simulink model "gm_uc3_preparation1_2017"  (R2018a)
settings: Solver=FixedStepDiscrete  StartTime=0.0  StopTime=0.6  FixedStep=2e-5  RelTol=1e-3  EnableMultiTasking=on
libraries: hdlsllib x6, simulink x3
(part 1 of 2)
settings Model: Creator=elahifah16  LastModifiedBy=Talha Rao
settings SolverCC: PositivePriorityOrder=on
settings OptimizationCC: BlockReduction=off  ConditionallyExecuteInputs=off  DefaultUnderspecifiedDataType=single  PassReuseOutputArgsAs=Individual arguments  MaxStackSize=64
settings DebuggingCC: InheritedTsInSrcMsg=none  ParameterTunabilityLossMsg=error  BusObjectLabelMismatch=error
settings HardwareCC: ProdBitPerPointer=32  ProdBitPerSizeT=32  ProdBitPerPtrDiffT=32  ProdLargestAtomicInteger=Long  ProdLargestAtomicFloat=Double  ProdWordSize=32  ProdHWDeviceType=ARM Compatible->ARM Cortex
settings SFSimCC: MATLABDynamicMemAlloc=off
settings RTWCC: SystemTargetFile=ert.tlc  HardwareBoard=Xilinx Zynq-7000 based board  TLCOptions="-aInlineSetEventsForThisBaseRateFcn=TLC_FALSE -aSuppressMultiTaskScheduler=TLC_FALSE  -aRateBasedStepFcn=0"  GenCodeOnly=on  TemplateMakefile=ert_default_tmf  GenerateReport=on  Toolchain=Xilinx Software Development Kit (SDK)  IncludeHyperlinkInReport=on  LaunchReport=on  GenerateTraceInfo=on  GenerateTraceReport=on  GenerateTraceReportSl=on  GenerateTraceReportSf=on  GenerateTraceReportEml=on  GenerateCodeReplacementReport=on
settings CodeAppCC: ForceParamTrailComments=on  IgnoreCustomStorageClasses=off  OperatorAnnotations=on  SimulinkDataObjDesc=on  SFDataObjDesc=on  InsertBlockDesc=on  StateflowObjectComments=on
settings ERTTargetCC: CodeReplacementLibrary=GNU C99 extensions  SupportComplex=off  SupportVariableSizeSignals=on  ExtModeTransport=1  ExtModeMexFile=ext_serial_win32_comm  MultiInstanceErrorCode=None  RootIOFormat=Structure reference

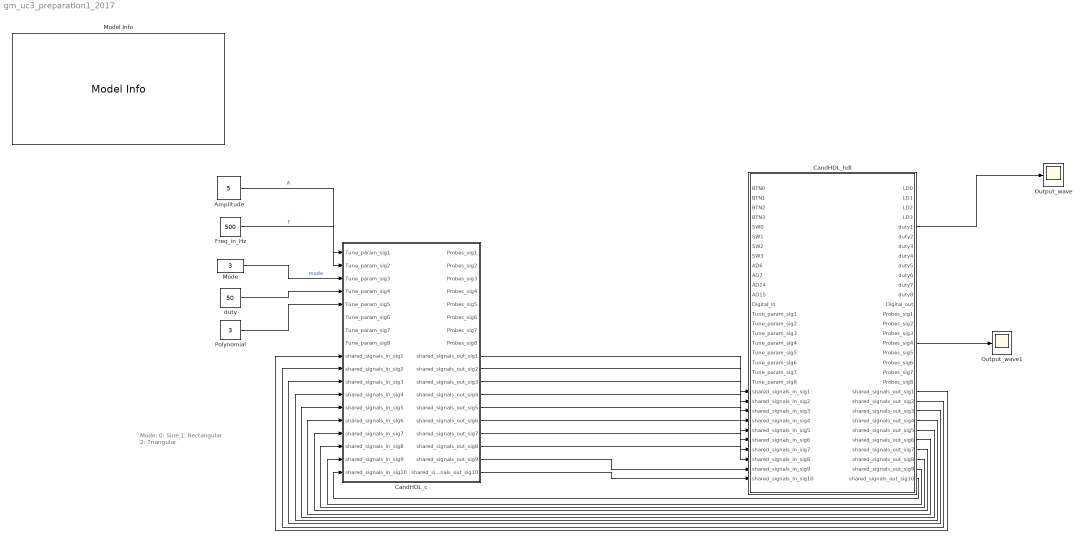
== system gm_uc3_preparation1_2017 ==
  note: Mode:
      | 0: Sine
      | 1: Rectangular
      | 2: Triangular
  Amplitude : Constant  Value=5  OutDataTypeStr=int32
  CandHDL_c : Subsystem  AncestorBlock=code_gen_library/CandHDL_c
  CandHDL_hdl : Subsystem
  Freq_in_Hz : Constant  Value=500  OutDataTypeStr=int32
  Mode : Constant  Value=3  OutDataTypeStr=int32
  Model Info : simulink/Model-Wide Utilities/Model Info  Frame=on  DisplayStringWithTags=|  HorizontalTextAlignment=Left  LeftAlignmentValue=0.02
      | Model Info
      | Creator:       R. Estrada, FH JOANNEUM, 2018
      | Modified by: %<ModifiedBy>
      | Modify Date: %<ModifiedDate>
      | Version:%<ModelVersion>
      | Description:
      | %<Description>
  Output_wave : Scope
  Output_wave1 : Scope
  Polynomial : Constant  Value=3  OutDataTypeStr=int32
  duty : Constant  Value=50  VectorParams1D=off  OutDataTypeStr=int32
  wires:
  CandHDL_hdl/17(Probes_sig4) -> Output_wave1/1
  Mode/1 -> CandHDL_c/3(Tune_param_sig3)  "mode"
  Freq_in_Hz/1 -> CandHDL_c/2(Tune_param_sig2)  "f"
  Polynomial/1 -> CandHDL_c/5(Tune_param_sig5)
  Amplitude/1 -> CandHDL_c/1(Tune_param_sig1)  "A"
  duty/1 -> CandHDL_c/4(Tune_param_sig4)
  CandHDL_hdl/31(shared_signals_out_sig10) -> CandHDL_c/18(shared_signals_in_sig10)
  CandHDL_c/18(shared_signals_out_sig10) -> CandHDL_hdl/31(shared_signals_in_sig10)
  CandHDL_hdl/30(shared_signals_out_sig9) -> CandHDL_c/17(shared_signals_in_sig9)
  CandHDL_c/17(shared_signals_out_sig9) -> CandHDL_hdl/30(shared_signals_in_sig9)
  CandHDL_hdl/29(shared_signals_out_sig8) -> CandHDL_c/16(shared_signals_in_sig8)
  CandHDL_c/16(shared_signals_out_sig8) -> CandHDL_hdl/29(shared_signals_in_sig8)
  CandHDL_hdl/28(shared_signals_out_sig7) -> CandHDL_c/15(shared_signals_in_sig7)
  CandHDL_c/15(shared_signals_out_sig7) -> CandHDL_hdl/28(shared_signals_in_sig7)
  CandHDL_hdl/27(shared_signals_out_sig6) -> CandHDL_c/14(shared_signals_in_sig6)
  CandHDL_c/14(shared_signals_out_sig6) -> CandHDL_hdl/27(shared_signals_in_sig6)
  CandHDL_hdl/26(shared_signals_out_sig5) -> CandHDL_c/13(shared_signals_in_sig5)
  CandHDL_c/13(shared_signals_out_sig5) -> CandHDL_hdl/26(shared_signals_in_sig5)
  CandHDL_hdl/25(shared_signals_out_sig4) -> CandHDL_c/12(shared_signals_in_sig4)
  CandHDL_c/12(shared_signals_out_sig4) -> CandHDL_hdl/25(shared_signals_in_sig4)
  CandHDL_hdl/24(shared_signals_out_sig3) -> CandHDL_c/11(shared_signals_in_sig3)
  CandHDL_c/11(shared_signals_out_sig3) -> CandHDL_hdl/24(shared_signals_in_sig3)
  CandHDL_hdl/23(shared_signals_out_sig2) -> CandHDL_c/10(shared_signals_in_sig2)
  CandHDL_c/10(shared_signals_out_sig2) -> CandHDL_hdl/23(shared_signals_in_sig2)
  CandHDL_hdl/22(shared_signals_out_sig1) -> CandHDL_c/9(shared_signals_in_sig1)
  CandHDL_c/9(shared_signals_out_sig1) -> CandHDL_hdl/22(shared_signals_in_sig1)
  CandHDL_hdl/5(duty1) -> Output_wave/1

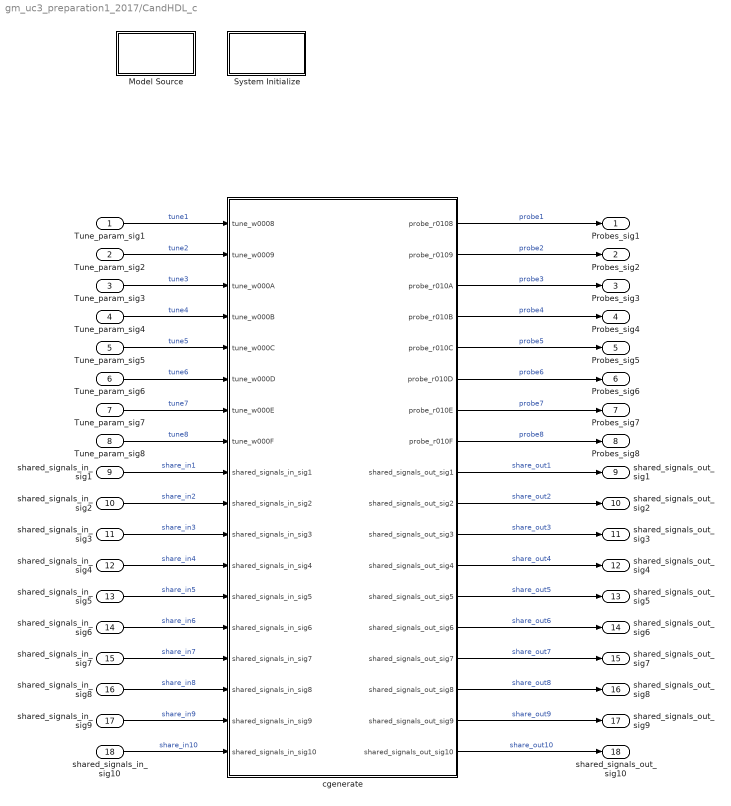
== system gm_uc3_preparation1_2017/CandHDL_c ==
  Tune_param_sig1 : Inport  OutDataTypeStr=int32
  Tune_param_sig2 : Inport  Port=2  OutDataTypeStr=int32
  Tune_param_sig3 : Inport  Port=3  OutDataTypeStr=int32
  Tune_param_sig4 : Inport  Port=4  OutDataTypeStr=int32
  Tune_param_sig5 : Inport  Port=5  OutDataTypeStr=int32
  Tune_param_sig6 : Inport  Port=6  OutDataTypeStr=int32
  Tune_param_sig7 : Inport  Port=7  OutDataTypeStr=int32
  Tune_param_sig8 : Inport  Port=8  OutDataTypeStr=int32
  shared_signals_in_sig1 : Inport  Port=9  OutDataTypeStr=int32
  shared_signals_in_sig2 : Inport  Port=10  OutDataTypeStr=int32
  shared_signals_in_sig3 : Inport  Port=11  OutDataTypeStr=int32
  shared_signals_in_sig4 : Inport  Port=12  OutDataTypeStr=int32
  shared_signals_in_sig5 : Inport  Port=13  OutDataTypeStr=int32
  shared_signals_in_sig6 : Inport  Port=14  OutDataTypeStr=int32
  shared_signals_in_sig7 : Inport  Port=15  OutDataTypeStr=int32
  shared_signals_in_sig8 : Inport  Port=16  OutDataTypeStr=int32
  shared_signals_in_sig9 : Inport  Port=17  OutDataTypeStr=int32
  shared_signals_in_sig10 : Inport  Port=18  OutDataTypeStr=int32
  Model Source : Subsystem  mask(Model Source){ShowInLibBrowser=0}
      mask prompts: ShowInLibBrowser "Simulink:masks:CustCodeMaskParam1_MP"
      settings: CopyFcn=cccopyfcn(gcb)  OpenFcn=ccopenfcn('Model Source')
      mask Help: eval('feval(''rtwprivate'',''rtwhelpview'',''rtw_model_source_block'')');
      mask Display: disp('Model\nSource');
  System Initialize : Subsystem  mask(System Initialize){ShowInLibBrowser=0}
      mask prompts: ShowInLibBrowser "Simulink:masks:CustCodeMaskParam1_MP"
      settings: CopyFcn=cccopyfcn(gcb)  OpenFcn=ccopenfcn('System Initialize Function')
      mask Help: eval('feval(''rtwprivate'',''rtwhelpview'',''rtw_sys_initialize_block'')');
      mask Display: disp('System\nInitialize');
  cgenerate : Subsystem
  Probes_sig1 : Outport  OutDataTypeStr=int32
  Probes_sig2 : Outport  Port=2  OutDataTypeStr=int32
  Probes_sig3 : Outport  Port=3  OutDataTypeStr=int32
  Probes_sig4 : Outport  Port=4  OutDataTypeStr=int32
  Probes_sig5 : Outport  Port=5  OutDataTypeStr=int32
  Probes_sig6 : Outport  Port=6  OutDataTypeStr=int32
  Probes_sig7 : Outport  Port=7  OutDataTypeStr=int32
  Probes_sig8 : Outport  Port=8  OutDataTypeStr=int32
  shared_signals_out_sig1 : Outport  Port=9  OutDataTypeStr=int32
  shared_signals_out_sig2 : Outport  Port=10  OutDataTypeStr=int32
  shared_signals_out_sig3 : Outport  Port=11  OutDataTypeStr=int32
  shared_signals_out_sig4 : Outport  Port=12  OutDataTypeStr=int32
  shared_signals_out_sig5 : Outport  Port=13  OutDataTypeStr=int32
  shared_signals_out_sig6 : Outport  Port=14  OutDataTypeStr=int32
  shared_signals_out_sig7 : Outport  Port=15  OutDataTypeStr=int32
  shared_signals_out_sig8 : Outport  Port=16  OutDataTypeStr=int32
  shared_signals_out_sig9 : Outport  Port=17  OutDataTypeStr=int32
  shared_signals_out_sig10 : Outport  Port=18  OutDataTypeStr=int32
  wires:
  cgenerate/18(shared_signals_out_sig10) -> shared_signals_out_sig10/1  "share_out10"
  cgenerate/17(shared_signals_out_sig9) -> shared_signals_out_sig9/1  "share_out9"
  cgenerate/16(shared_signals_out_sig8) -> shared_signals_out_sig8/1  "share_out8"
  cgenerate/15(shared_signals_out_sig7) -> shared_signals_out_sig7/1  "share_out7"
  cgenerate/14(shared_signals_out_sig6) -> shared_signals_out_sig6/1  "share_out6"
  cgenerate/13(shared_signals_out_sig5) -> shared_signals_out_sig5/1  "share_out5"
  cgenerate/12(shared_signals_out_sig4) -> shared_signals_out_sig4/1  "share_out4"
  cgenerate/11(shared_signals_out_sig3) -> shared_signals_out_sig3/1  "share_out3"
  cgenerate/10(shared_signals_out_sig2) -> shared_signals_out_sig2/1  "share_out2"
  cgenerate/9(shared_signals_out_sig1) -> shared_signals_out_sig1/1  "share_out1"
  shared_signals_in_sig10/1 -> cgenerate/18(shared_signals_in_sig10)  "share_in10"
  shared_signals_in_sig9/1 -> cgenerate/17(shared_signals_in_sig9)  "share_in9"
  shared_signals_in_sig8/1 -> cgenerate/16(shared_signals_in_sig8)  "share_in8"
  shared_signals_in_sig7/1 -> cgenerate/15(shared_signals_in_sig7)  "share_in7"
  shared_signals_in_sig6/1 -> cgenerate/14(shared_signals_in_sig6)  "share_in6"
  shared_signals_in_sig5/1 -> cgenerate/13(shared_signals_in_sig5)  "share_in5"
  shared_signals_in_sig4/1 -> cgenerate/12(shared_signals_in_sig4)  "share_in4"
  shared_signals_in_sig3/1 -> cgenerate/11(shared_signals_in_sig3)  "share_in3"
  shared_signals_in_sig2/1 -> cgenerate/10(shared_signals_in_sig2)  "share_in2"
  shared_signals_in_sig1/1 -> cgenerate/9(shared_signals_in_sig1)  "share_in1"
  Tune_param_sig8/1 -> cgenerate/8(tune_w000F)  "tune8"
  Tune_param_sig7/1 -> cgenerate/7(tune_w000E)  "tune7"
  Tune_param_sig6/1 -> cgenerate/6(tune_w000D)  "tune6"
  Tune_param_sig5/1 -> cgenerate/5(tune_w000C)  "tune5"
  Tune_param_sig4/1 -> cgenerate/4(tune_w000B)  "tune4"
  Tune_param_sig3/1 -> cgenerate/3(tune_w000A)  "tune3"
  Tune_param_sig2/1 -> cgenerate/2(tune_w0009)  "tune2"
  Tune_param_sig1/1 -> cgenerate/1(tune_w0008)  "tune1"
  cgenerate/8(probe_r010F) -> Probes_sig8/1  "probe8"
  cgenerate/7(probe_r010E) -> Probes_sig7/1  "probe7"
  cgenerate/6(probe_r010D) -> Probes_sig6/1  "probe6"
  cgenerate/5(probe_r010C) -> Probes_sig5/1  "probe5"
  cgenerate/4(probe_r010B) -> Probes_sig4/1  "probe4"
  cgenerate/3(probe_r010A) -> Probes_sig3/1  "probe3"
  cgenerate/2(probe_r0109) -> Probes_sig2/1  "probe2"
  cgenerate/1(probe_r0108) -> Probes_sig1/1  "probe1"

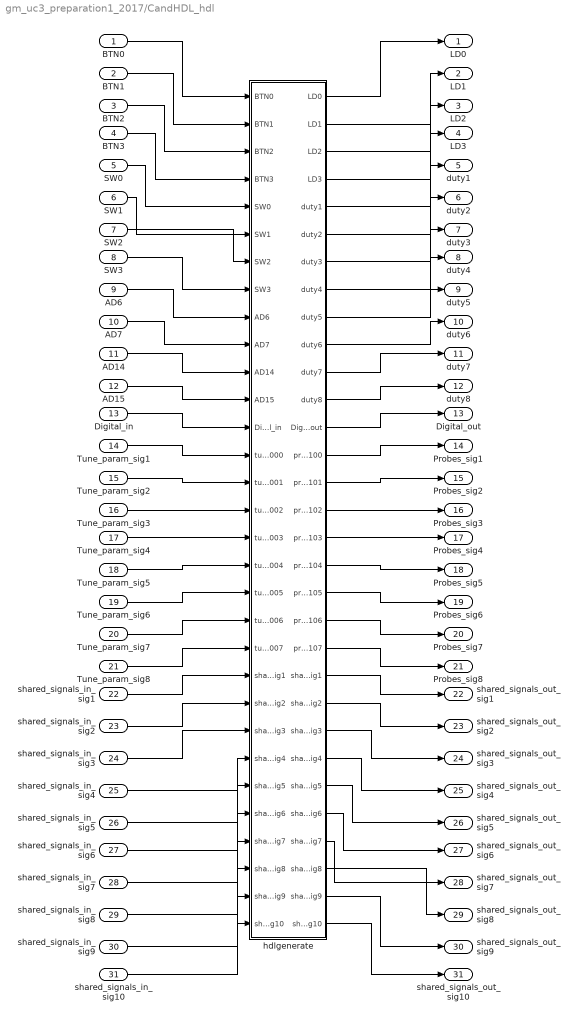
== system gm_uc3_preparation1_2017/CandHDL_hdl ==
  BTN0 : Inport  OutDataTypeStr=boolean  PortDimensions=1
  BTN1 : Inport  Port=2  OutDataTypeStr=boolean  PortDimensions=1
  BTN2 : Inport  Port=3  OutDataTypeStr=boolean  PortDimensions=1
  BTN3 : Inport  Port=4  OutDataTypeStr=boolean  PortDimensions=1
  SW0 : Inport  Port=5  OutDataTypeStr=boolean  PortDimensions=1
  SW1 : Inport  Port=6  OutDataTypeStr=boolean  PortDimensions=1
  SW2 : Inport  Port=7  OutDataTypeStr=boolean  PortDimensions=1
  SW3 : Inport  Port=8  OutDataTypeStr=boolean  PortDimensions=1
  AD6 : Inport  Port=9  OutDataTypeStr=uint16  PortDimensions=1
  AD7 : Inport  Port=10  OutDataTypeStr=uint16  PortDimensions=1
  AD14 : Inport  Port=11  OutDataTypeStr=uint16  PortDimensions=1
  AD15 : Inport  Port=12  OutDataTypeStr=uint16  PortDimensions=1
  Digital_in : Inport  Port=13  OutDataTypeStr=uint8  PortDimensions=1
  Tune_param_sig1 : Inport  Port=14  OutDataTypeStr=int32  PortDimensions=1
  Tune_param_sig2 : Inport  Port=15  OutDataTypeStr=int32  PortDimensions=1
  Tune_param_sig3 : Inport  Port=16  OutDataTypeStr=int32  PortDimensions=1
  Tune_param_sig4 : Inport  Port=17  OutDataTypeStr=int32  PortDimensions=1
  Tune_param_sig5 : Inport  Port=18  OutDataTypeStr=int32  PortDimensions=1
  Tune_param_sig6 : Inport  Port=19  OutDataTypeStr=int32  PortDimensions=1
  Tune_param_sig7 : Inport  Port=20  OutDataTypeStr=int32  PortDimensions=1
  Tune_param_sig8 : Inport  Port=21  OutDataTypeStr=int32  PortDimensions=1
  shared_signals_in_sig1 : Inport  Port=22  OutDataTypeStr=int32  PortDimensions=1
  shared_signals_in_sig2 : Inport  Port=23  OutDataTypeStr=int32  PortDimensions=1  SampleTime=2e-05
  shared_signals_in_sig3 : Inport  Port=24  OutDataTypeStr=int32  PortDimensions=1  SampleTime=2e-05
  shared_signals_in_sig4 : Inport  Port=25  OutDataTypeStr=int32  PortDimensions=1  SampleTime=2e-05
  shared_signals_in_sig5 : Inport  Port=26  OutDataTypeStr=int32  PortDimensions=1  SampleTime=2e-05
  shared_signals_in_sig6 : Inport  Port=27  OutDataTypeStr=int32  PortDimensions=1  SampleTime=2e-05
  shared_signals_in_sig7 : Inport  Port=28  OutDataTypeStr=int32  PortDimensions=1
  shared_signals_in_sig8 : Inport  Port=29  OutDataTypeStr=int32  PortDimensions=1  SampleTime=2e-05
  shared_signals_in_sig9 : Inport  Port=30  OutDataTypeStr=int32  PortDimensions=1
  shared_signals_in_sig10 : Inport  Port=31  OutDataTypeStr=int32  PortDimensions=1
  hdlgenerate : Subsystem
  LD0 : Outport  OutDataTypeStr=boolean
  LD1 : Outport  Port=2  OutDataTypeStr=boolean
  LD2 : Outport  Port=3  OutDataTypeStr=boolean
  LD3 : Outport  Port=4  OutDataTypeStr=boolean
  duty1 : Outport  Port=5  OutDataTypeStr=uint16
  duty2 : Outport  Port=6  OutDataTypeStr=uint16
  duty3 : Outport  Port=7  OutDataTypeStr=uint16
  duty4 : Outport  Port=8  OutDataTypeStr=uint16
  duty5 : Outport  Port=9  OutDataTypeStr=uint16
  duty6 : Outport  Port=10  OutDataTypeStr=uint16
  duty7 : Outport  Port=11  OutDataTypeStr=uint16
  duty8 : Outport  Port=12  OutDataTypeStr=uint16
  Digital_out : Outport  Port=13  OutDataTypeStr=uint8
  Probes_sig1 : Outport  Port=14  OutDataTypeStr=int32
  Probes_sig2 : Outport  Port=15  OutDataTypeStr=int32
  Probes_sig3 : Outport  Port=16  OutDataTypeStr=int32
  Probes_sig4 : Outport  Port=17  OutDataTypeStr=int32
  Probes_sig5 : Outport  Port=18  OutDataTypeStr=int32
  Probes_sig6 : Outport  Port=19  OutDataTypeStr=int32
  Probes_sig7 : Outport  Port=20  OutDataTypeStr=int32
  Probes_sig8 : Outport  Port=21  OutDataTypeStr=int32
  shared_signals_out_sig1 : Outport  Port=22  OutDataTypeStr=int32
  shared_signals_out_sig2 : Outport  Port=23  OutDataTypeStr=int32
  shared_signals_out_sig3 : Outport  Port=24  OutDataTypeStr=int32
  shared_signals_out_sig4 : Outport  Port=25  OutDataTypeStr=int32
  shared_signals_out_sig5 : Outport  Port=26  OutDataTypeStr=int32
  shared_signals_out_sig6 : Outport  Port=27  OutDataTypeStr=int32
  shared_signals_out_sig7 : Outport  Port=28  OutDataTypeStr=int32
  shared_signals_out_sig8 : Outport  Port=29  OutDataTypeStr=int32
  shared_signals_out_sig9 : Outport  Port=30  OutDataTypeStr=int32
  shared_signals_out_sig10 : Outport  Port=31  OutDataTypeStr=int32
  wires:
  BTN0/1 -> hdlgenerate/1(BTN0)
  BTN1/1 -> hdlgenerate/2(BTN1)
  BTN2/1 -> hdlgenerate/3(BTN2)
  BTN3/1 -> hdlgenerate/4(BTN3)
  SW0/1 -> hdlgenerate/5(SW0)
  SW1/1 -> hdlgenerate/6(SW1)
  SW2/1 -> hdlgenerate/7(SW2)
  SW3/1 -> hdlgenerate/8(SW3)
  AD6/1 -> hdlgenerate/9(AD6)
  AD7/1 -> hdlgenerate/10(AD7)
  AD14/1 -> hdlgenerate/11(AD14)
  AD15/1 -> hdlgenerate/12(AD15)
  Digital_in/1 -> hdlgenerate/13(Digital_in)
  Tune_param_sig1/1 -> hdlgenerate/14(tune_w0000)
  Tune_param_sig2/1 -> hdlgenerate/15(tune_w0001)
  Tune_param_sig3/1 -> hdlgenerate/16(tune_w0002)
  Tune_param_sig4/1 -> hdlgenerate/17(tune_w0003)
  Tune_param_sig5/1 -> hdlgenerate/18(tune_w0004)
  Tune_param_sig6/1 -> hdlgenerate/19(tune_w0005)
  Tune_param_sig7/1 -> hdlgenerate/20(tune_w0006)
  Tune_param_sig8/1 -> hdlgenerate/21(tune_w0007)
  shared_signals_in_sig1/1 -> hdlgenerate/22(shared_signals_in_sig1)
  shared_signals_in_sig2/1 -> hdlgenerate/23(shared_signals_in_sig2)
  shared_signals_in_sig3/1 -> hdlgenerate/24(shared_signals_in_sig3)
  shared_signals_in_sig4/1 -> hdlgenerate/25(shared_signals_in_sig4)
  shared_signals_in_sig5/1 -> hdlgenerate/26(shared_signals_in_sig5)
  shared_signals_in_sig6/1 -> hdlgenerate/27(shared_signals_in_sig6)
  shared_signals_in_sig7/1 -> hdlgenerate/28(shared_signals_in_sig7)
  shared_signals_in_sig8/1 -> hdlgenerate/29(shared_signals_in_sig8)
  shared_signals_in_sig9/1 -> hdlgenerate/30(shared_signals_in_sig9)
  shared_signals_in_sig10/1 -> hdlgenerate/31(shared_signals_in_sig10)
  hdlgenerate/1(LD0) -> LD0/1
  hdlgenerate/2(LD1) -> LD1/1
  hdlgenerate/3(LD2) -> LD2/1
  hdlgenerate/4(LD3) -> LD3/1
  hdlgenerate/5(duty1) -> duty1/1
  hdlgenerate/6(duty2) -> duty2/1
  hdlgenerate/7(duty3) -> duty3/1
  hdlgenerate/8(duty4) -> duty4/1
  hdlgenerate/9(duty5) -> duty5/1
  hdlgenerate/10(duty6) -> duty6/1
  hdlgenerate/11(duty7) -> duty7/1
  hdlgenerate/12(duty8) -> duty8/1
  hdlgenerate/13(Digital_out) -> Digital_out/1
  hdlgenerate/14(probe_r0100) -> Probes_sig1/1
  hdlgenerate/15(probe_r0101) -> Probes_sig2/1
  hdlgenerate/16(probe_r0102) -> Probes_sig3/1
  hdlgenerate/17(probe_r0103) -> Probes_sig4/1
  hdlgenerate/18(probe_r0104) -> Probes_sig5/1
  hdlgenerate/19(probe_r0105) -> Probes_sig6/1
  hdlgenerate/20(probe_r0106) -> Probes_sig7/1
  hdlgenerate/21(probe_r0107) -> Probes_sig8/1
  hdlgenerate/22(shared_signals_out_sig1) -> shared_signals_out_sig1/1
  hdlgenerate/23(shared_signals_out_sig2) -> shared_signals_out_sig2/1
  hdlgenerate/24(shared_signals_out_sig3) -> shared_signals_out_sig3/1
  hdlgenerate/25(shared_signals_out_sig4) -> shared_signals_out_sig4/1
  hdlgenerate/26(shared_signals_out_sig5) -> shared_signals_out_sig5/1
  hdlgenerate/27(shared_signals_out_sig6) -> shared_signals_out_sig6/1
  hdlgenerate/28(shared_signals_out_sig7) -> shared_signals_out_sig7/1
  hdlgenerate/29(shared_signals_out_sig8) -> shared_signals_out_sig8/1
  hdlgenerate/30(shared_signals_out_sig9) -> shared_signals_out_sig9/1
  hdlgenerate/31(shared_signals_out_sig10) -> shared_signals_out_sig10/1

== system gm_uc3_preparation1_2017/CandHDL_c/Model Source ==

== system gm_uc3_preparation1_2017/CandHDL_c/System Initialize ==

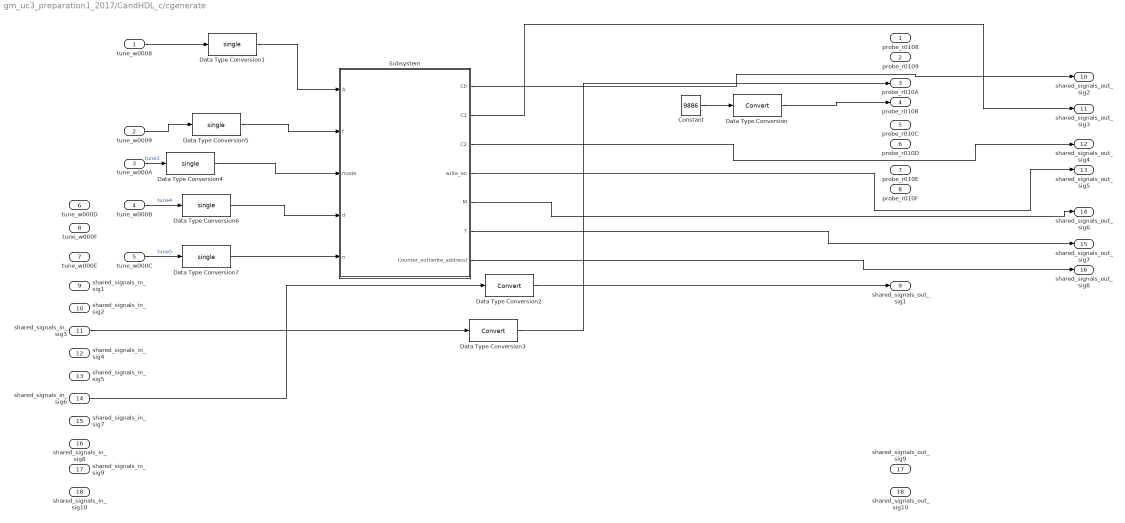
== system gm_uc3_preparation1_2017/CandHDL_c/cgenerate ==
  tune_w0008 : Inport  OutDataTypeStr=int32
  tune_w0009 : Inport  Port=2  OutDataTypeStr=int32
  tune_w000A : Inport  Port=3  OutDataTypeStr=int32
  tune_w000B : Inport  Port=4  OutDataTypeStr=int32
  tune_w000C : Inport  Port=5  OutDataTypeStr=int32
  tune_w000D : Inport  Port=6  OutDataTypeStr=int32
  tune_w000E : Inport  Port=7  OutDataTypeStr=int32
  tune_w000F : Inport  Port=8  OutDataTypeStr=int32
  shared_signals_in_sig1 : Inport  Port=9  OutDataTypeStr=int32
  shared_signals_in_sig2 : Inport  Port=10  OutDataTypeStr=int32
  shared_signals_in_sig3 : Inport  Port=11  OutDataTypeStr=int32
  shared_signals_in_sig4 : Inport  Port=12  OutDataTypeStr=int32
  shared_signals_in_sig5 : Inport  Port=13  OutDataTypeStr=int32
  shared_signals_in_sig6 : Inport  Port=14  OutDataTypeStr=int32
  shared_signals_in_sig7 : Inport  Port=15  OutDataTypeStr=int32
  shared_signals_in_sig8 : Inport  Port=16  OutDataTypeStr=int32
  shared_signals_in_sig9 : Inport  Port=17  OutDataTypeStr=int32
  shared_signals_in_sig10 : Inport  Port=18  OutDataTypeStr=int32
  Constant : Constant  Value=9886  OutDataTypeStr=int16  SampleTime=-1
  Data Type Conversion : DataTypeConversion
  Data Type Conversion{1,4..7} (5 alike) : DataTypeConversion  OutDataTypeStr=single
  Data Type Conversion2 : DataTypeConversion
  Data Type Conversion3 : DataTypeConversion
  Subsystem : Subsystem
  probe_r0108 : Outport  OutDataTypeStr=int32
  probe_r0109 : Outport  Port=2  OutDataTypeStr=int32
  probe_r010A : Outport  Port=3  OutDataTypeStr=int32
  probe_r010B : Outport  Port=4  OutDataTypeStr=int32
  probe_r010C : Outport  Port=5  OutDataTypeStr=int32
  probe_r010D : Outport  Port=6  OutDataTypeStr=int32
  probe_r010E : Outport  Port=7  OutDataTypeStr=int32
  probe_r010F : Outport  Port=8  OutDataTypeStr=int32
  shared_signals_out_sig1 : Outport  Port=9  OutDataTypeStr=int32
  shared_signals_out_sig2 : Outport  Port=10  OutDataTypeStr=int32
  shared_signals_out_sig3 : Outport  Port=11  OutDataTypeStr=int32
  shared_signals_out_sig4 : Outport  Port=12  OutDataTypeStr=int32
  shared_signals_out_sig5 : Outport  Port=13  OutDataTypeStr=int32
  shared_signals_out_sig6 : Outport  Port=14  OutDataTypeStr=int32
  shared_signals_out_sig7 : Outport  Port=15  OutDataTypeStr=int32
  shared_signals_out_sig8 : Outport  Port=16  OutDataTypeStr=int32
  shared_signals_out_sig9 : Outport  Port=17  OutDataTypeStr=int32
  shared_signals_out_sig10 : Outport  Port=18  OutDataTypeStr=int32
  wires:
  Data Type Conversion7/1 -> Subsystem/5(n)
  Data Type Conversion6/1 -> Subsystem/4(d)
  Data Type Conversion4/1 -> Subsystem/3(mode)
  Data Type Conversion5/1 -> Subsystem/2("f ")
  Data Type Conversion1/1 -> Subsystem/1(A)
  Subsystem/7(Counter_out(write_address)) -> shared_signals_out_sig8/1
  Subsystem/6(T) -> shared_signals_out_sig7/1
  Subsystem/4(write_en) -> shared_signals_out_sig5/1
  Subsystem/3(C2) -> shared_signals_out_sig4/1
  Subsystem/2(C1) -> shared_signals_out_sig3/1
  Subsystem/5(M) -> shared_signals_out_sig6/1
  Subsystem/1(C0) -> shared_signals_out_sig2/1
  tune_w000B/1 -> Data Type Conversion6/1  "tune4"
  tune_w000A/1 -> Data Type Conversion4/1  "tune3"
  tune_w0009/1 -> Data Type Conversion5/1
  shared_signals_in_sig6/1 -> Data Type Conversion2/1
  tune_w0008/1 -> Data Type Conversion1/1
  tune_w000C/1 -> Data Type Conversion7/1  "tune5"
  Data Type Conversion3/1 -> probe_r010A/1
  Data Type Conversion2/1 -> shared_signals_out_sig1/1
  shared_signals_in_sig3/1 -> Data Type Conversion3/1
  Data Type Conversion/1 -> probe_r010B/1
  Constant/1 -> Data Type Conversion/1

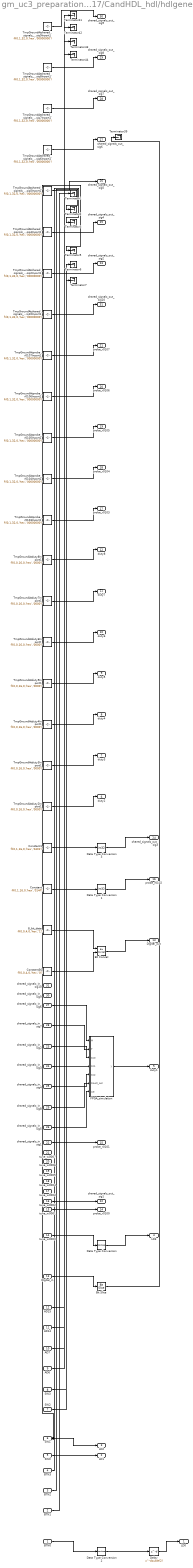
== system gm_uc3_preparation1_2017/CandHDL_hdl/hdlgenerate ==
  BTN0 : Inport  OutDataTypeStr=boolean  PortDimensions=1
  BTN1 : Inport  Port=2  OutDataTypeStr=boolean  PortDimensions=1
  BTN2 : Inport  Port=3  OutDataTypeStr=boolean  PortDimensions=1
  BTN3 : Inport  Port=4  OutDataTypeStr=boolean  PortDimensions=1
  SW0 : Inport  Port=5  OutDataTypeStr=boolean  PortDimensions=1
  SW1 : Inport  Port=6  OutDataTypeStr=boolean  PortDimensions=1
  SW2 : Inport  Port=7  OutDataTypeStr=boolean  PortDimensions=1
  SW3 : Inport  Port=8  OutDataTypeStr=boolean  PortDimensions=1
  AD6 : Inport  Port=9  OutDataTypeStr=uint16  PortDimensions=1
  AD7 : Inport  Port=10  OutDataTypeStr=uint16  PortDimensions=1
  AD14 : Inport  Port=11  OutDataTypeStr=uint16  PortDimensions=1
  AD15 : Inport  Port=12  OutDataTypeStr=uint16  PortDimensions=1
  Digital_in : Inport  Port=13  OutDataTypeStr=uint8  PortDimensions=1
  tune_w0000 : Inport  Port=14  OutDataTypeStr=int32  PortDimensions=1
  tune_w0001 : Inport  Port=15  OutDataTypeStr=int32  PortDimensions=1
  tune_w0002 : Inport  Port=16  OutDataTypeStr=int32  PortDimensions=1
  tune_w0003 : Inport  Port=17  OutDataTypeStr=int32  PortDimensions=1
  tune_w0004 : Inport  Port=18  OutDataTypeStr=int32  PortDimensions=1
  tune_w0005 : Inport  Port=19  OutDataTypeStr=int32  PortDimensions=1
  tune_w0006 : Inport  Port=20  OutDataTypeStr=int32  PortDimensions=1
  tune_w0007 : Inport  Port=21  OutDataTypeStr=int32  PortDimensions=1
  shared_signals_in_sig1 : Inport  Port=22  OutDataTypeStr=int32  PortDimensions=1
  shared_signals_in_sig2 : Inport  Port=23  OutDataTypeStr=int32  PortDimensions=1  SampleTime=2e-05
  shared_signals_in_sig3 : Inport  Port=24  OutDataTypeStr=int32  PortDimensions=1  SampleTime=2e-05
  shared_signals_in_sig4 : Inport  Port=25  OutDataTypeStr=int32  PortDimensions=1  SampleTime=2e-05
  shared_signals_in_sig5 : Inport  Port=26  OutDataTypeStr=int32  PortDimensions=1  SampleTime=2e-05
  shared_signals_in_sig6 : Inport  Port=27  OutDataTypeStr=int32  PortDimensions=1  SampleTime=2e-05
  shared_signals_in_sig7 : Inport  Port=28  OutDataTypeStr=int32  PortDimensions=1
  shared_signals_in_sig8 : Inport  Port=29  OutDataTypeStr=int32  PortDimensions=1  SampleTime=2e-05
  shared_signals_in_sig9 : Inport  Port=30  OutDataTypeStr=int32  PortDimensions=1
  shared_signals_in_sig10 : Inport  Port=31  OutDataTypeStr=int32  PortDimensions=1
  8_bit_data : Constant  Value=fi(0,0,4,0,'hex','1')  OutDataTypeStr=fixdt(0, 4, 0)  SampleTime=-1
  Bit Concat : hdlsllib/Logic and Bit Operations/Bit Concat  numInputs=2
      settings: SourceProductName=HDL Coder  SourceProductBaseCode=HD
  Bit Slice : hdlsllib/Logic and Bit Operations/Bit Slice  lidx=double(0)  ridx=double(0)
  Constant : Constant  Value=fi(0,1,16,0,'hex','014f')  OutDataTypeStr=int16  SampleTime=-1
  Constant1 : Constant  Value=fi(0,1,16,0,'hex','0401')  OutDataTypeStr=int16  SampleTime=-1
  Constant36 : Constant  Value=fi(0,0,4,0,'hex','0')  OutDataTypeStr=fixdt(0, 4, 0)  SampleTime=-1
  Data Type Conversion : DataTypeConversion  OutDataTypeStr=boolean
  Data Type Conversion1 : DataTypeConversion  OutDataTypeStr=int32  SampleTime=2e-05
  Data Type Conversion2 : DataTypeConversion  OutDataTypeStr=boolean
  Data Type Conversion3 : DataTypeConversion  OutDataTypeStr=int32  SampleTime=2e-05
  Delay : Delay  DelayLength=double(2)  InitialCondition=0  InputProcessing=Inherited  SampleTime=2e-05
  FPGA_simulation : Subsystem
  Terminator{1..3,5..7,39,41..44} (11 alike) : Terminator
  TmpGroundAtduty2Inport1 : Constant  Value=fi(0,0,16,0,'hex','0000')  VectorParams1D=off  OutDataTypeStr=uint16  SampleTime=-1
  TmpGroundAtduty3Inport1 : Constant  Value=fi(0,0,16,0,'hex','0000')  VectorParams1D=off  OutDataTypeStr=uint16  SampleTime=-1
  TmpGroundAtduty4Inport1 : Constant  Value=fi(0,0,16,0,'hex','0000')  VectorParams1D=off  OutDataTypeStr=uint16  SampleTime=-1
  TmpGroundAtduty5Inport1 : Constant  Value=fi(0,0,16,0,'hex','0000')  VectorParams1D=off  OutDataTypeStr=uint16  SampleTime=-1
  TmpGroundAtduty6Inport1 : Constant  Value=fi(0,0,16,0,'hex','0000')  VectorParams1D=off  OutDataTypeStr=uint16  SampleTime=-1
  TmpGroundAtduty7Inport1 : Constant  Value=fi(0,0,16,0,'hex','0000')  VectorParams1D=off  OutDataTypeStr=uint16  SampleTime=-1
  TmpGroundAtduty8Inport1 : Constant  Value=fi(0,0,16,0,'hex','0000')  VectorParams1D=off  OutDataTypeStr=uint16  SampleTime=-1
  TmpGroundAtprobe_r0103Inport1 : Constant  Value=fi(0,1,32,0,'hex','00000000')  VectorParams1D=off  OutDataTypeStr=int32  SampleTime=-1
  TmpGroundAtprobe_r0104Inport1 : Constant  Value=fi(0,1,32,0,'hex','00000000')  VectorParams1D=off  OutDataTypeStr=int32  SampleTime=-1
  TmpGroundAtprobe_r0105Inport1 : Constant  Value=fi(0,1,32,0,'hex','00000000')  VectorParams1D=off  OutDataTypeStr=int32  SampleTime=-1
  TmpGroundAtprobe_r0106Inport1 : Constant  Value=fi(0,1,32,0,'hex','00000000')  VectorParams1D=off  OutDataTypeStr=int32  SampleTime=-1
  TmpGroundAtprobe_r0107Inport1 : Constant  Value=fi(0,1,32,0,'hex','00000000')  VectorParams1D=off  OutDataTypeStr=int32  SampleTime=-1
  TmpGroundAtshared_signals_out_sig10Inport1 : Constant  Value=fi(0,1,32,0,'hex','00000000')  VectorParams1D=off  OutDataTypeStr=int32  SampleTime=-1
  TmpGroundAtshared_signals_out_sig2Inport1 : Constant  Value=fi(0,1,32,0,'hex','00000000')  VectorParams1D=off  OutDataTypeStr=int32  SampleTime=-1
  TmpGroundAtshared_signals_out_sig4Inport1 : Constant  Value=fi(0,1,32,0,'hex','00000000')  VectorParams1D=off  OutDataTypeStr=int32  SampleTime=-1
  TmpGroundAtshared_signals_out_sig5Inport1 : Constant  Value=fi(0,1,32,0,'hex','00000000')  VectorParams1D=off  OutDataTypeStr=int32  SampleTime=-1
  TmpGroundAtshared_signals_out_sig6Inport1 : Constant  Value=fi(0,1,32,0,'hex','00000000')  VectorParams1D=off  OutDataTypeStr=int32  SampleTime=-1
  TmpGroundAtshared_signals_out_sig7Inport1 : Constant  Value=fi(0,1,32,0,'hex','00000000')  VectorParams1D=off  OutDataTypeStr=int32  SampleTime=-1
  TmpGroundAtshared_signals_out_sig8Inport1 : Constant  Value=fi(0,1,32,0,'hex','00000000')  VectorParams1D=off  OutDataTypeStr=int32  SampleTime=-1
  TmpGroundAtshared_signals_out_sig9Inport1 : Constant  Value=fi(0,1,32,0,'hex','00000000')  VectorParams1D=off  OutDataTypeStr=int32  SampleTime=-1
  LD0 : Outport  OutDataTypeStr=boolean
  LD1 : Outport  Port=2  OutDataTypeStr=boolean
  LD2 : Outport  Port=3  OutDataTypeStr=boolean
  LD3 : Outport  Port=4  OutDataTypeStr=boolean
  duty1 : Outport  Port=5  OutDataTypeStr=uint16
  duty2 : Outport  Port=6  OutDataTypeStr=uint16
  duty3 : Outport  Port=7  OutDataTypeStr=uint16
  duty4 : Outport  Port=8  OutDataTypeStr=uint16
  duty5 : Outport  Port=9  OutDataTypeStr=uint16
  duty6 : Outport  Port=10  OutDataTypeStr=uint16
  duty7 : Outport  Port=11  OutDataTypeStr=uint16
  duty8 : Outport  Port=12  OutDataTypeStr=uint16
  Digital_out : Outport  Port=13  OutDataTypeStr=uint8
  probe_r0100 : Outport  Port=14  OutDataTypeStr=int32
  probe_r0101 : Outport  Port=15  OutDataTypeStr=int32
  probe_r0102 : Outport  Port=16  OutDataTypeStr=int32
  probe_r0103 : Outport  Port=17  OutDataTypeStr=int32
  probe_r0104 : Outport  Port=18  OutDataTypeStr=int32
  probe_r0105 : Outport  Port=19  OutDataTypeStr=int32
  probe_r0106 : Outport  Port=20  OutDataTypeStr=int32
  probe_r0107 : Outport  Port=21  OutDataTypeStr=int32
  shared_signals_out_sig1 : Outport  Port=22  OutDataTypeStr=int32
  shared_signals_out_sig2 : Outport  Port=23  OutDataTypeStr=int32
  shared_signals_out_sig3 : Outport  Port=24  OutDataTypeStr=int32
  shared_signals_out_sig4 : Outport  Port=25  OutDataTypeStr=int32
  shared_signals_out_sig5 : Outport  Port=26  OutDataTypeStr=int32
  shared_signals_out_sig6 : Outport  Port=27  OutDataTypeStr=int32
  shared_signals_out_sig7 : Outport  Port=28  OutDataTypeStr=int32
  shared_signals_out_sig8 : Outport  Port=29  OutDataTypeStr=int32
  shared_signals_out_sig9 : Outport  Port=30  OutDataTypeStr=int32
  shared_signals_out_sig10 : Outport  Port=31  OutDataTypeStr=int32
  wires:
  BTN0/1 -> Data Type Conversion2/1
  BTN1/1 -> Terminator1/1
  BTN2/1 -> Terminator2/1
  BTN3/1 -> Terminator3/1
  SW0/1 -> LD1/1
  SW1/1 -> Terminator5/1, LD2/1
  SW2/1 -> Terminator6/1
  SW3/1 -> Terminator7/1
  AD6/1 -> Terminator41/1
  AD7/1 -> Terminator42/1
  AD14/1 -> Terminator43/1
  AD15/1 -> Terminator44/1
  Digital_in/1 -> Bit Slice/1
  tune_w0000/1 -> Data Type Conversion/1
  tune_w0001/1 -> probe_r0100/1
  tune_w0002/1 -> shared_signals_out_sig1/1
  shared_signals_in_sig1/1 -> probe_r0101/1
  shared_signals_in_sig2/1 -> FPGA_simulation/3(Cc0)
  shared_signals_in_sig3/1 -> FPGA_simulation/4(Cc1)
  shared_signals_in_sig4/1 -> FPGA_simulation/5(Cc2)
  shared_signals_in_sig5/1 -> FPGA_simulation/7(we)
  shared_signals_in_sig6/1 -> FPGA_simulation/1(M)
  shared_signals_in_sig7/1 -> FPGA_simulation/2(T)
  shared_signals_in_sig8/1 -> FPGA_simulation/6(Count_out)
  8_bit_data/1 -> Bit Concat/1
  Bit Concat/1 -> Digital_out/1
  Bit Slice/1 -> Terminator39/1
  Constant/1 -> Data Type Conversion1/1
  Constant1/1 -> Data Type Conversion3/1
  Constant36/1 -> Bit Concat/2
  Data Type Conversion/1 -> LD3/1
  Data Type Conversion1/1 -> probe_r0102/1
  Data Type Conversion2/1 -> Delay/1
  Data Type Conversion3/1 -> shared_signals_out_sig3/1
  Delay/1 -> LD0/1
  FPGA_simulation/1(y) -> duty1/1
  TmpGroundAtduty2Inport1/1 -> duty2/1
  TmpGroundAtduty3Inport1/1 -> duty3/1
  TmpGroundAtduty4Inport1/1 -> duty4/1
  TmpGroundAtduty5Inport1/1 -> duty5/1
  TmpGroundAtduty6Inport1/1 -> duty6/1
  TmpGroundAtduty7Inport1/1 -> duty7/1
  TmpGroundAtduty8Inport1/1 -> duty8/1
  TmpGroundAtprobe_r0103Inport1/1 -> probe_r0103/1
  TmpGroundAtprobe_r0104Inport1/1 -> probe_r0104/1
  TmpGroundAtprobe_r0105Inport1/1 -> probe_r0105/1
  TmpGroundAtprobe_r0106Inport1/1 -> probe_r0106/1
  TmpGroundAtprobe_r0107Inport1/1 -> probe_r0107/1
  TmpGroundAtshared_signals_out_sig10Inport1/1 -> shared_signals_out_sig10/1
  TmpGroundAtshared_signals_out_sig2Inport1/1 -> shared_signals_out_sig2/1
  TmpGroundAtshared_signals_out_sig4Inport1/1 -> shared_signals_out_sig4/1
  TmpGroundAtshared_signals_out_sig5Inport1/1 -> shared_signals_out_sig5/1
  TmpGroundAtshared_signals_out_sig6Inport1/1 -> shared_signals_out_sig6/1
  TmpGroundAtshared_signals_out_sig7Inport1/1 -> shared_signals_out_sig7/1
  TmpGroundAtshared_signals_out_sig8Inport1/1 -> shared_signals_out_sig8/1
  TmpGroundAtshared_signals_out_sig9Inport1/1 -> shared_signals_out_sig9/1

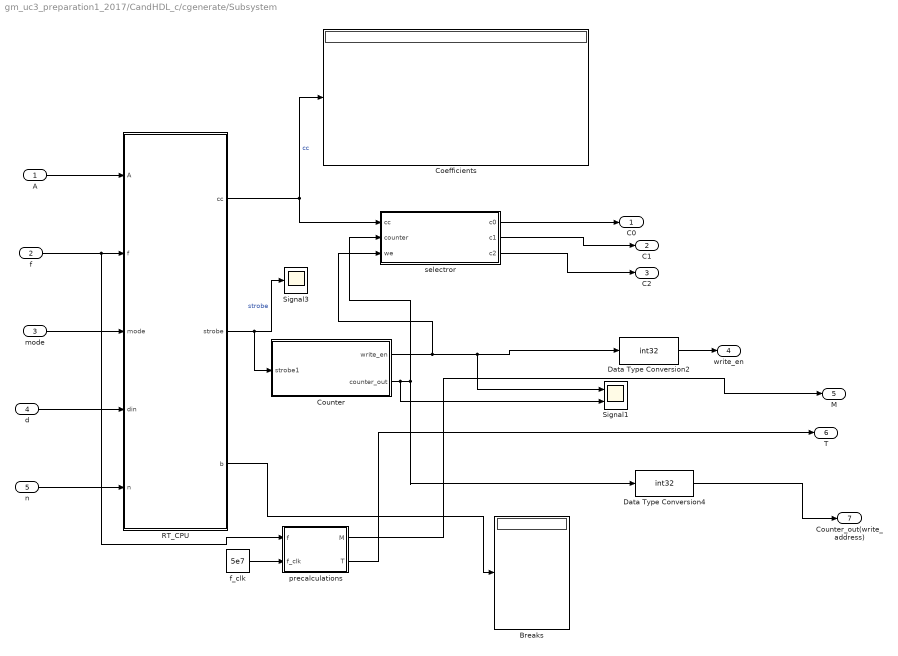
== system gm_uc3_preparation1_2017/CandHDL_c/cgenerate/Subsystem ==
  A : Inport  OutDataTypeStr=single
  "f " : Inport  Port=2  OutDataTypeStr=single
  mode : Inport  Port=3  OutDataTypeStr=single
  d : Inport  Port=4  OutDataTypeStr=single
  n : Inport  Port=5  OutDataTypeStr=single
  Breaks : Display
  Coefficients : Display
  Counter : Subsystem  TreatAsAtomicUnit=on
  Data Type Conversion2 : DataTypeConversion  OutDataTypeStr=int32
  Data Type Conversion4 : DataTypeConversion  OutDataTypeStr=int32
  RT_CPU : MATLAB Function  TreatAsAtomicUnit=on
  Signal1 : Scope  NumInputPorts=2
  Signal3 : Scope
  f_clk : Constant  Value=5e7  OutDataTypeStr=int32
  precalculations : Subsystem
  selectror : Subsystem  TreatAsAtomicUnit=on
  C0 : Outport  OutDataTypeStr=int32
  C1 : Outport  Port=2  OutDataTypeStr=int32
  C2 : Outport  Port=3  OutDataTypeStr=int32
  write_en : Outport  Port=4  OutDataTypeStr=int32
  M : Outport  Port=5  OutDataTypeStr=int32
  T : Outport  Port=6  OutDataTypeStr=int32
  Counter_out(write_address) : Outport  Port=7  OutDataTypeStr=int32
  wires:
  Data Type Conversion4/1 -> Counter_out(write_address)/1
  mode/1 -> RT_CPU/3(mode)
  f_clk/1 -> precalculations/2(f_clk)
  d/1 -> RT_CPU/4(din)
  RT_CPU/3(b) -> Breaks/1
  RT_CPU/2(strobe) -> Signal3/1, Counter/1(strobe1)  "strobe"
  n/1 -> RT_CPU/5(n)
  Counter/2(counter_out) -> Signal1/2, Data Type Conversion4/1, selectror/2(counter)
  RT_CPU/1(cc) -> Coefficients/1, selectror/1(cc)  "cc"
  "f "/1 -> RT_CPU/2(f), precalculations/1(f)
  Counter/1(write_en) -> Data Type Conversion2/1, Signal1/1, selectror/3(we)
  A/1 -> RT_CPU/1(A)
  selectror/3(c2) -> C2/1
  selectror/1(c0) -> C0/1
  precalculations/2(T) -> T/1
  precalculations/1(M) -> M/1
  Data Type Conversion2/1 -> write_en/1
  selectror/2(c1) -> C1/1

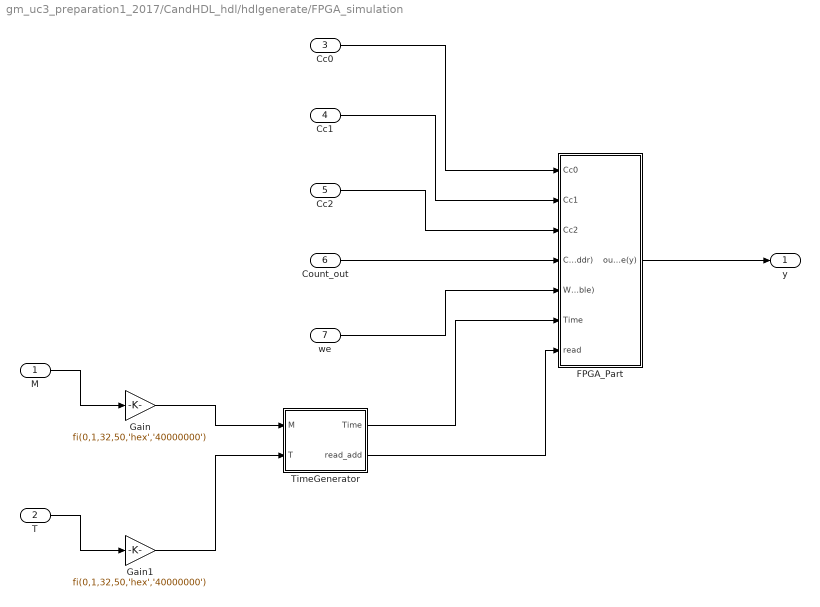
== system gm_uc3_preparation1_2017/CandHDL_hdl/hdlgenerate/FPGA_simulation ==
  M : Inport  PortDimensions=1  SampleTime=2e-05
  T : Inport  Port=2  PortDimensions=1
  Cc0 : Inport  Port=3  PortDimensions=1  SampleTime=2e-05
  Cc1 : Inport  Port=4  PortDimensions=1  SampleTime=2e-05
  Cc2 : Inport  Port=5  PortDimensions=1  SampleTime=2e-05
  Count_out : Inport  Port=6  PortDimensions=1  SampleTime=2e-05
  we : Inport  Port=7  PortDimensions=1  SampleTime=2e-05
  " FPGA_Part" : Subsystem
  Gain : Gain  Gain=fi(0,1,32,50,'hex','40000000')  ParamDataTypeStr=fixdt(1, 32, 50)  OutDataTypeStr=fixdt(1, 32, 19)  SampleTime=2e-05
  Gain1 : Gain  Gain=fi(0,1,32,50,'hex','40000000')  ParamDataTypeStr=fixdt(1, 32, 50)  OutDataTypeStr=fixdt(1, 32, 19)
  TimeGenerator : Subsystem
  y : Outport
  wires:
  M/1 -> Gain/1
  T/1 -> Gain1/1
  Cc0/1 -> " FPGA_Part"/1(Cc0)
  Cc1/1 -> " FPGA_Part"/2(Cc1)
  Cc2/1 -> " FPGA_Part"/3(Cc2)
  Count_out/1 -> " FPGA_Part"/4(Counter_out(write_addr))
  we/1 -> " FPGA_Part"/5(We(write_enable))
  " FPGA_Part"/1(output_wave(y)) -> y/1
  Gain/1 -> TimeGenerator/1(M)
  Gain1/1 -> TimeGenerator/2(T)
  TimeGenerator/1(Time) -> " FPGA_Part"/6(Time)
  TimeGenerator/2(read_add) -> " FPGA_Part"/7(read)

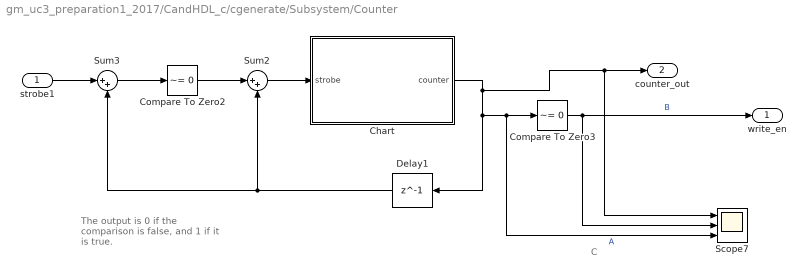
== system gm_uc3_preparation1_2017/CandHDL_c/cgenerate/Subsystem/Counter ==
  note: C
  note: The output is 0 if the comparison is false, and 1 if it is true.
  strobe1 : Inport
  Chart : Stateflow chart  TreatAsAtomicUnit=on
  Compare To Zero2 : simulink/Logic and Bit Operations/Compare To Zero  relop=~=  OutDataTypeStr=boolean
  Compare To Zero3 : simulink/Logic and Bit Operations/Compare To Zero  relop=~=  OutDataTypeStr=boolean
  Delay1 : Delay  DelayLength=1
  Scope7 : Scope  NumInputPorts=3
  Sum2 : Sum  Inputs=|++  OutDataTypeStr=single
  Sum3 : Sum  Inputs=|++  OutDataTypeStr=single
  write_en : Outport
  counter_out : Outport  Port=2
  wires:
  Compare To Zero3/1 -> write_en/1, Scope7/2  "B"
  strobe1/1 -> Sum3/1
  Chart/1(counter) -> Delay1/1, Compare To Zero3/1, Scope7/3, counter_out/1, Scope7/1  "A"
  Sum2/1 -> Chart/1(strobe)
  Delay1/1 -> Sum3/2, Sum2/2
  Sum3/1 -> Compare To Zero2/1
  Compare To Zero2/1 -> Sum2/1

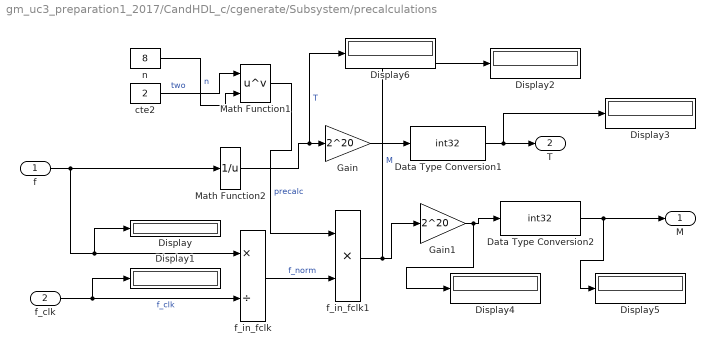
== system gm_uc3_preparation1_2017/CandHDL_c/cgenerate/Subsystem/precalculations ==
  f : Inport
  f_clk : Inport  Port=2
  Data Type Conversion1 : DataTypeConversion  OutDataTypeStr=int32
  Data Type Conversion2 : DataTypeConversion  OutDataTypeStr=int32
  Display{,1..6} (7 alike) : Display
  Gain : Gain  Gain=2^20  OutDataTypeStr=single
  Gain1 : Gain  Gain=2^20  OutDataTypeStr=single
  Math Function1 : Math  Operator=pow  SaturateOnIntegerOverflow=on
  Math Function2 : Math  Operator=reciprocal  OutDataTypeStr=single  SaturateOnIntegerOverflow=on
  cte2 : Constant  Value=2  OutDataTypeStr=single  SampleTime=-1
  f_in_fclk : Product  Inputs=*/  OutDataTypeStr=single
  f_in_fclk1 : Product  Inputs=**  OutDataTypeStr=single
  n : Constant  Value=8  OutDataTypeStr=single  SampleTime=-1
  M : Outport
  T : Outport  Port=2
  wires:
  Gain1/1 -> Data Type Conversion2/1, Display4/1
  Gain/1 -> Data Type Conversion1/1
  Data Type Conversion2/1 -> M/1, Display5/1
  f_in_fclk1/1 -> Gain1/1, Display2/1  "M"
  Data Type Conversion1/1 -> T/1, Display3/1
  f/1 -> f_in_fclk/1, Display/1, Math Function2/1
  f_in_fclk/1 -> f_in_fclk1/2  "f_norm"
  f_clk/1 -> Display1/1, f_in_fclk/2  "f_clk"
  Math Function2/1 -> Gain/1, Display6/1  "T"
  Math Function1/1 -> f_in_fclk1/1  "precalc"
  n/1 -> Math Function1/2  "n"
  cte2/1 -> Math Function1/1  "two"

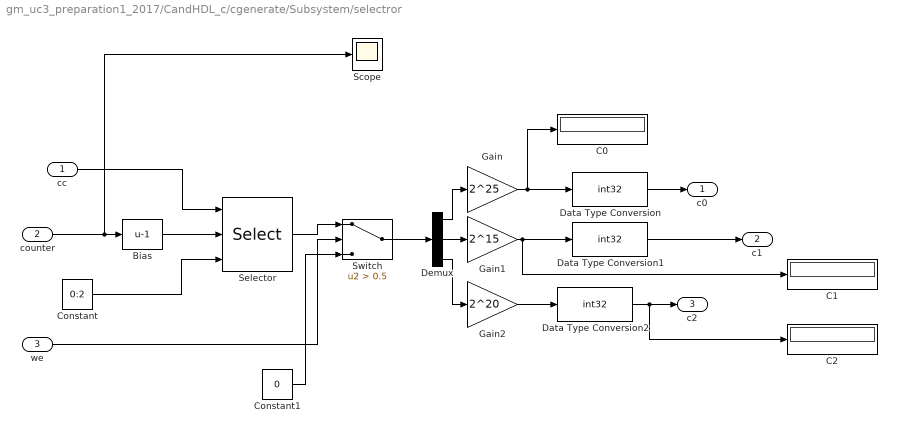
== system gm_uc3_preparation1_2017/CandHDL_c/cgenerate/Subsystem/selectror ==
  cc : Inport
  counter : Inport  Port=2
  we : Inport  Port=3
  Bias : Bias  Bias=-1
  C0 : Display
  C1 : Display
  C2 : Display
  Constant : Constant  Value=0:2  OutDataTypeStr=single
  Constant1 : Constant  Value=0  OutDataTypeStr=single
  Data Type Conversion : DataTypeConversion  OutDataTypeStr=int32
  Data Type Conversion1 : DataTypeConversion  OutDataTypeStr=int32
  Data Type Conversion2 : DataTypeConversion  OutDataTypeStr=int32
  Demux : Demux  Outputs=3
  Gain : Gain  Gain=2^25  OutDataTypeStr=single
  Gain1 : Gain  Gain=2^15  OutDataTypeStr=single
  Gain2 : Gain  Gain=2^20  OutDataTypeStr=single
  Scope : Scope
  Selector : Selector  NumberOfDimensions=2  IndexMode=Zero-based  InputPortWidth=3  IndexOptions=Index vector (port),Index vector (port)  Indices=[1 3],1  OutputSizes=1,1
  Switch : Switch  Criteria=u2 > Threshold  Threshold=0.5  OutDataTypeStr=single
  c0 : Outport
  c1 : Outport  Port=2
  c2 : Outport  Port=3
  wires:
  Bias/1 -> Selector/2
  Constant1/1 -> Switch/3
  we/1 -> Switch/2
  Selector/1 -> Switch/1
  Switch/1 -> Demux/1
  counter/1 -> Scope/1, Bias/1
  Demux/3 -> Gain2/1
  Gain2/1 -> Data Type Conversion2/1
  Demux/2 -> Gain1/1
  Gain1/1 -> C1/1, Data Type Conversion1/1
  Demux/1 -> Gain/1
  Gain/1 -> Data Type Conversion/1, C0/1
  Data Type Conversion2/1 -> c2/1, C2/1
  Data Type Conversion1/1 -> c1/1
  Data Type Conversion/1 -> c0/1
  Constant/1 -> Selector/3
  cc/1 -> Selector/1

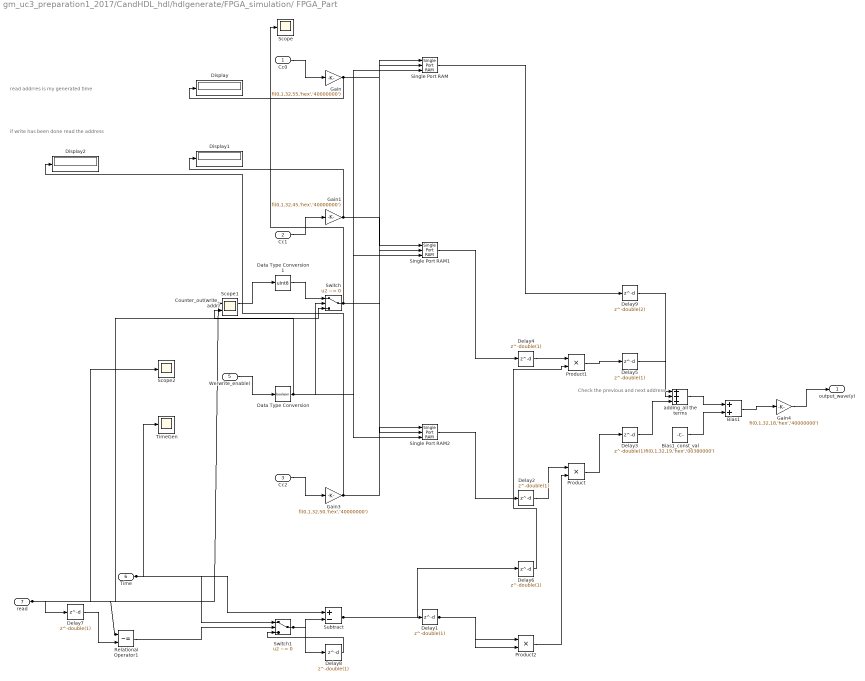
== system gm_uc3_preparation1_2017/CandHDL_hdl/hdlgenerate/FPGA_simulation/ FPGA_Part ==
  note: read addrres is my generated time
  note: if write has been done read the address
  note: Check the previous and next address
  Cc0 : Inport  PortDimensions=1  SampleTime=2e-05
  Cc1 : Inport  Port=2  PortDimensions=1  SampleTime=2e-05
  Cc2 : Inport  Port=3  PortDimensions=1  SampleTime=2e-05
  Counter_out(write_addr) : Inport  Port=4  PortDimensions=1  SampleTime=2e-05
  We(write_enable) : Inport  Port=5  PortDimensions=1  SampleTime=2e-05
  Time : Inport  Port=6  PortDimensions=1  SampleTime=2e-05
  read : Inport  Port=7  PortDimensions=1  SampleTime=2e-05
  Bias1 : Sum  AccumDataTypeStr=fixdt(1, 32, 19)  OutDataTypeStr=fixdt(1, 32, 19)  RndMeth=Nearest  SampleTime=2e-05
  Bias1_const_val : Constant  Value=fi(0,1,32,19,'hex','00380000')  VectorParams1D=off  OutDataTypeStr=fixdt(1, 32, 19)  SampleTime=-1
  Data Type Conversion : DataTypeConversion  OutDataTypeStr=boolean  SampleTime=2e-05
  Data Type Conversion1 : DataTypeConversion  OutDataTypeStr=uint8  SampleTime=2e-05
  Delay{1..8} (8 alike) : Delay  DelayLength=double(1)  InitialCondition=0  InputProcessing=Inherited  SampleTime=2e-05
  Delay9 : Delay  DelayLength=double(2)  InitialCondition=0  InputProcessing=Inherited  SampleTime=2e-05
  Display : Display
  Display1 : Display
  Display2 : Display
  Gain : Gain  Gain=fi(0,1,32,55,'hex','40000000')  ParamDataTypeStr=fixdt(1, 32, 55)  OutDataTypeStr=fixdt(1, 32, 19)  SampleTime=2e-05
  Gain1 : Gain  Gain=fi(0,1,32,45,'hex','40000000')  ParamDataTypeStr=fixdt(1, 32, 45)  OutDataTypeStr=fixdt(1, 32, 19)  SampleTime=2e-05
  Gain3 : Gain  Gain=fi(0,1,32,50,'hex','40000000')  ParamDataTypeStr=fixdt(1, 32, 50)  OutDataTypeStr=fixdt(1, 32, 19)  SampleTime=2e-05
  Gain4 : Gain  Gain=fi(0,1,32,18,'hex','40000000')  ParamDataTypeStr=fixdt(1, 32, 18)  OutDataTypeStr=uint16  SampleTime=2e-05
  Product : Product  Inputs=**  OutDataTypeStr=fixdt(1, 32, 19)  SampleTime=2e-05
  Product1 : Product  Inputs=**  OutDataTypeStr=fixdt(1, 32, 19)  SampleTime=2e-05
  Product2 : Product  Inputs=**  OutDataTypeStr=fixdt(1, 32, 19)  SampleTime=2e-05
  Relational Operator1 : RelationalOperator  Operator=~=  OutDataTypeStr=boolean  SampleTime=2e-05  RndMeth=Nearest
  Scope : Scope
  Scope1 : Scope  NumInputPorts=2
  Scope2 : Scope
  Single Port RAM : hdlsllib/HDL RAMs/Single Port RAM  ram_size=8  dout_type=Old data
      settings: SourceProductName=HDL Coder  SourceProductBaseCode=HD
  Single Port RAM1 : hdlsllib/HDL RAMs/Single Port RAM  ram_size=8  dout_type=Old data
      settings: SourceProductName=HDL Coder  SourceProductBaseCode=HD
  Single Port RAM2 : hdlsllib/HDL RAMs/Single Port RAM  ram_size=8  dout_type=Old data
      settings: SourceProductName=HDL Coder  SourceProductBaseCode=HD
  Subtract : Sum  Inputs=+-  AccumDataTypeStr=fixdt(1, 32, 19)  OutDataTypeStr=fixdt(1, 32, 19)  SampleTime=2e-05
  Switch : Switch  Criteria=u2 ~= 0  Threshold=double(0)  OutDataTypeStr=uint8  SampleTime=2e-05
  Switch1 : Switch  Criteria=u2 ~= 0  Threshold=double(0)  OutDataTypeStr=fixdt(1, 32, 19)  SampleTime=2e-05
  TimeGen : Scope
  adding_all the terms : Sum  Inputs=+++  AccumDataTypeStr=fixdt(1, 32, 19)  OutDataTypeStr=fixdt(1, 32, 19)  SampleTime=2e-05
  output_wave(y) : Outport
  wires:
  Cc0/1 -> Gain/1
  Cc1/1 -> Gain1/1
  Cc2/1 -> Gain3/1
  Counter_out(write_addr)/1 -> Data Type Conversion1/1
  We(write_enable)/1 -> Data Type Conversion/1
  Time/1 -> Switch1/1, Subtract/1, TimeGen/1
  read/1 -> Switch/3, Relational Operator1/1, Scope2/1, Scope1/1, Delay7/1
  Bias1/1 -> Gain4/1
  Data Type Conversion/1 -> Switch/2, Scope1/2, Single Port RAM/3, Single Port RAM1/3, Single Port RAM2/3
  Data Type Conversion1/1 -> Switch/1
  Delay1/1 -> Product2/2, Product2/1
  Delay2/1 -> Product/1
  Delay3/1 -> adding_all the terms/3
  Delay4/1 -> Product1/1
  Delay5/1 -> adding_all the terms/2
  Delay6/1 -> Product1/2
  Delay7/1 -> Relational Operator1/2
  Delay8/1 -> Switch1/3
  Delay9/1 -> adding_all the terms/1
  Gain/1 -> Display/1, Single Port RAM/1
  Gain1/1 -> Display1/1, Single Port RAM1/1
  Gain3/1 -> Display2/1, Single Port RAM2/1
  Gain4/1 -> output_wave(y)/1
  Product/1 -> Delay3/1
  Product1/1 -> Delay5/1
  Product2/1 -> Product/2
  Relational Operator1/1 -> Switch1/2
  Single Port RAM/1 -> Delay9/1
  Single Port RAM1/1 -> Delay4/1
  Single Port RAM2/1 -> Delay2/1
  Subtract/1 -> Delay6/1, Delay1/1
  Switch/1 -> Scope/1, Single Port RAM/2, Single Port RAM1/2, Single Port RAM2/2
  Switch1/1 -> Subtract/2, Delay8/1
  adding_all the terms/1 -> Bias1/1
  Bias1_const_val/1 -> Bias1/2

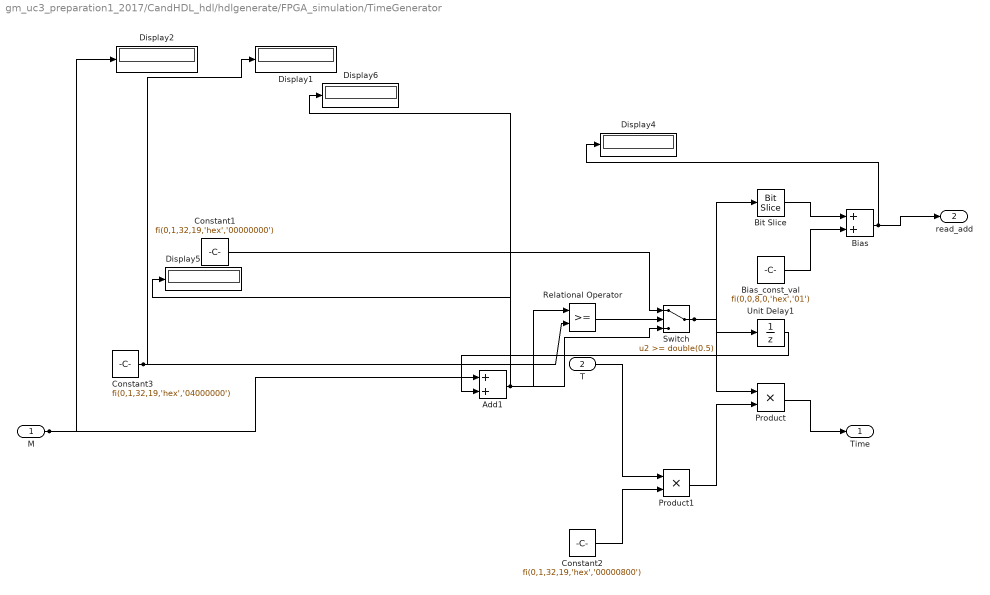
== system gm_uc3_preparation1_2017/CandHDL_hdl/hdlgenerate/FPGA_simulation/TimeGenerator ==
  M : Inport  OutDataTypeStr=fixdt(1,32,19)  PortDimensions=1  SampleTime=2e-05
  T : Inport  Port=2  OutDataTypeStr=fixdt(1,32,19)  PortDimensions=1
  Add1 : Sum  AccumDataTypeStr=fixdt(1, 32, 19)  OutDataTypeStr=fixdt(1, 32, 19)  SampleTime=2e-05
  Bias : Sum  AccumDataTypeStr=uint8  OutDataTypeStr=uint8  RndMeth=Nearest  SampleTime=2e-05
  Bias_const_val : Constant  Value=fi(0,0,8,0,'hex','01')  VectorParams1D=off  OutDataTypeStr=uint8  SampleTime=-1
  Bit Slice : hdlsllib/Logic and Bit Operations/Bit Slice  lidx=double(26)  ridx=double(19)
  Constant1 : Constant  Value=fi(0,1,32,19,'hex','00000000')  OutDataTypeStr=fixdt(1, 32, 19)  SampleTime=-1
  Constant2 : Constant  Value=fi(0,1,32,19,'hex','00000800')  OutDataTypeStr=fixdt(1, 32, 19)  SampleTime=-1
  Constant3 : Constant  Value=fi(0,1,32,19,'hex','04000000')  OutDataTypeStr=fixdt(1, 32, 19)  SampleTime=-1
  Display{1..2,4..6} (5 alike) : Display
  Product : Product  Inputs=**  OutDataTypeStr=fixdt(1, 32, 19)  SampleTime=2e-05
  Product1 : Product  Inputs=**  OutDataTypeStr=fixdt(1, 32, 19)
  Relational Operator : RelationalOperator  OutDataTypeStr=fixdt(1, 32, 19)  SampleTime=2e-05  RndMeth=Nearest
  Switch : Switch  Threshold=double(0.5)  OutDataTypeStr=fixdt(1, 32, 19)  SampleTime=2e-05
  Unit Delay1 : UnitDelay  InitialCondition=fi(0,1,32,19,'hex','00000000')  SampleTime=2e-05
  Time : Outport
  read_add : Outport  Port=2
  wires:
  M/1 -> Add1/1, Display2/1
  T/1 -> Product1/1
  Add1/1 -> Switch/3, Relational Operator/1, Display6/1, Display5/1
  Bias/1 -> Display4/1, read_add/1
  Bit Slice/1 -> Bias/1
  Constant1/1 -> Switch/1
  Constant2/1 -> Product1/2
  Constant3/1 -> Relational Operator/2, Display1/1
  Product/1 -> Time/1
  Product1/1 -> Product/2
  Relational Operator/1 -> Switch/2
  Switch/1 -> Product/1, Bit Slice/1, Unit Delay1/1
  Unit Delay1/1 -> Add1/2
  Bias_const_val/1 -> Bias/2

== stateflow chart gm_uc3_preparation1_2017/CandHDL_c/cgenerate/Subsystem/Counter/Chart ==
  settings: executeAtInitialization=1
  state sate2
    entry:
    strobe_temp=0;
    during:
    counter=0;
  state state1
    entry:
    strobe_temp=strobe;
    counter=0;
    during :
    counter=counter+1;
  (default) -> state1
  state1 -> sate2 : [(counter >128)]
  sate2 -> state1 : [(strobe==1)]
  data: strobe input single; counter output single; strobe_temp local single
